simulink model "autotransformerSubtractive"  (R2018a)
settings: Solver=VariableStepAuto  StartTime=0.0  StopTime=0.1  FixedStep=0.01666  RelTol=1e-4
values from neighbouring files (symbols this model uses):
  Freq = 60    [Autotransformer.m]    (also in transformer2wind.m; transformer3wind.m)
  k = 240/2400    (= 0.1)    [Autotransformer.m]    (also in transformer2wind.m)
  L1 = 0.92/(2*pi*Freq)    (= 0.00244037579408)    [Autotransformer.m]    (also in transformer2wind.m = 0.00119366207319; transformer3wind.m = 0.00119366207319)
  L2 = 0.009/(2*pi*Freq)    (= 2.38732414638e-05)    [Autotransformer.m]    (also in transformer2wind.m = 1.19366207319e-05; transformer3wind.m = 1.19366207319e-05)
  Ll = Xl/(2*pi*Freq)    (= 0.0202328075769)    [Autotransformer.m]    (also in transformer2wind.m = 0.000610160156975)
  Lo = 4370/(2*pi*Freq)    (= 11.5917850219)    [Autotransformer.m]    (also in transformer2wind.m = 4.11150269654; transformer3wind.m = 4.11150269654)
  R1 = 0.72    [Autotransformer.m]    (also in transformer2wind.m = 0.2; transformer3wind.m = 0.2)
  R2 = 0.007    [Autotransformer.m]    (also in transformer2wind.m = 0.002; transformer3wind.m = 0.002)
  Rl = 440000/(208*208)    (= 10.1701183432)    [Autotransformer.m]    (also in transformer2wind.m = 0.307480832)
  Ro = 632    [Autotransformer.m]    (also in transformer2wind.m = 10000; transformer3wind.m = 10000)
  S = 50000    [Autotransformer.m]    (also in transformer2wind.m = 150000; transformer3wind.m = 150000)
  V1 = 2400    [Autotransformer.m]    (also in transformer3wind.m)
  V2 = 240    [Autotransformer.m]    (also in transformer2wind.m; transformer3wind.m)
  Vs = 2405*sqrt(2)    [Autotransformer.m]    (also in transformer2wind.m = 2455*sqrt(2); transformer3wind.m = 2455*sqrt(2))
libraries: fl_lib x15, powerlib x9, nesl_utility x5
settings Model: Creator=Noor  LastModifiedBy=Noor

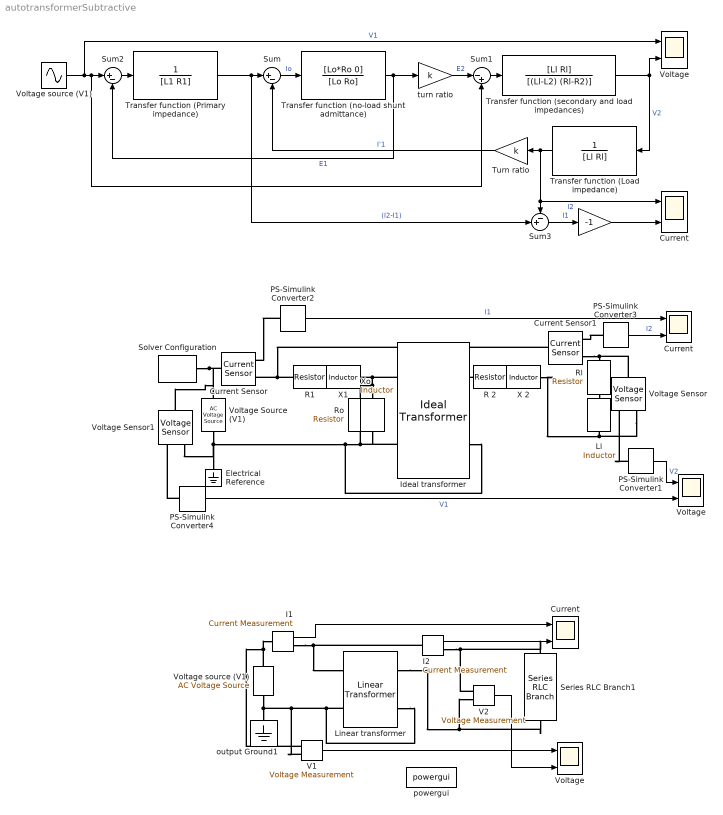
== system autotransformerSubtractive ==
  "  " : Gain  Gain=-1
  " Current" : Scope  NumInputPorts=2
  " Voltage" : Scope  NumInputPorts=2
  Current : Scope  NumInputPorts=2
  "Current " : Scope  NumInputPorts=2
  Current Sensor : fl_lib/Electrical/Electrical Sensors/Current Sensor
  Current Sensor1 : fl_lib/Electrical/Electrical Sensors/Current Sensor
  Electrical Reference : fl_lib/Electrical/Electrical Elements/Electrical Reference
  "I1 " : powerlib/Measurements/Current Measurement  Tag=PoWeRsYsTeMmEaSuReMeNt  PhasorSimulation=off  OutputType=Magnitude  PSBequivalent=0
  "I2 " : powerlib/Measurements/Current Measurement  Tag=PoWeRsYsTeMmEaSuReMeNt  PhasorSimulation=off  OutputType=Magnitude  PSBequivalent=0
  Ideal transformer : fl_lib/Electrical/Electrical Elements/Ideal Transformer  n=1/k  i1_specify=off  i1_priority=None  i1=0 A  i1_nominal_specify=off  i1_nominal_unit=A  i1_nominal_value=1  v1_specify=off  v1_priority=None  v1=0 V  v1_nominal_specify=off  v1_nominal_unit=V  v1_nominal_value=1  i2_specify=off  i2_priority=None  i2=0 A  i2_nominal_specify=off  i2_nominal_unit=A  i2_nominal_value=1  v2_specify=off  v2_priority=None  v2=0 V  v2_nominal_specify=off  v2_nominal_unit=V  v2_nominal_value=1
      settings: SourceProductName=Simscape  SourceProductBaseCode=SS
  Linear transformer : powerlib/Elements/Linear Transformer  UNITS=SI  NominalPower=[S Freq]  winding1=[V1 R1 L1]  winding2=[V2 R2 L2]  ThreeWindings=off  winding3=[3.15e+05 0.7938 0.084225]  RmLm=[Ro Lo]  Measurements=None  DataType=on
  Ll : fl_lib/Electrical/Electrical Elements/Inductor  l=Ll H  r=0 Ohm  g=0 1/Ohm  i_specify=off  i_priority=None  i=0 A  i_nominal_specify=off  i_nominal_unit=A  i_nominal_value=1  v_specify=off  v_priority=None  v=0 V  v_nominal_specify=off  v_nominal_unit=V  v_nominal_value=1  i_L_specify=off  i_L_priority=High  i_L=0 A  i_L_nominal_specify=off  i_L_nominal_unit=A  i_L_nominal_value=1
  PS-Simulink Converter{1..4} (4 alike) : nesl_utility/PS-Simulink Converter  PhysicalDomain=network_engine_domain  SubClassName=ps_output  LeftPortType=input  RightPortType=output  PseudoPeriodic=off  Frequencies=[]  Unit=1  AffineConversion=off
  R 2 : fl_lib/Electrical/Electrical Elements/Resistor  R=R2 Ohm  i_specify=off  i_priority=None  i=0 A  i_nominal_specify=off  i_nominal_unit=A  i_nominal_value=1  v_specify=off  v_priority=None  v=0 V  v_nominal_specify=off  v_nominal_unit=V  v_nominal_value=1
  R1 : fl_lib/Electrical/Electrical Elements/Resistor  R=R1 Ohm  i_specify=off  i_priority=None  i=0 A  i_nominal_specify=off  i_nominal_unit=A  i_nominal_value=1  v_specify=off  v_priority=None  v=0 V  v_nominal_specify=off  v_nominal_unit=V  v_nominal_value=1
  Rl : fl_lib/Electrical/Electrical Elements/Resistor  R=Rl Ohm  i_specify=off  i_priority=None  i=0 A  i_nominal_specify=off  i_nominal_unit=A  i_nominal_value=1  v_specify=off  v_priority=None  v=0 V  v_nominal_specify=off  v_nominal_unit=V  v_nominal_value=1
  Ro : fl_lib/Electrical/Electrical Elements/Resistor  R=Ro Ohm  i_specify=off  i_priority=None  i=0 A  i_nominal_specify=off  i_nominal_unit=A  i_nominal_value=1  v_specify=off  v_priority=None  v=0 V  v_nominal_specify=off  v_nominal_unit=V  v_nominal_value=1
  Series RLC Branch1 : powerlib/Elements/Series RLC Branch  LConnTagsString=__new0  RConnTagsString=__new0  BranchType=RL  Resistance=Rl  Inductance=Ll  SetiL0=off  InitialCurrent=0  Capacitance=1e-6  Setx0=off  InitialVoltage=0  Measurements=None
  Solver Configuration : nesl_utility/Solver Configuration  PhysicalDomain=network_engine_domain  SubClassName=solver  LeftPortType=input  RightPortType=generic  Tones=[]  Harmonics=[]  SimulateNoise=off  Profile=off  UseLocalSampling=off  EnableSwitchedLinearOptims=on  FrequencyDomain=off  UseCCode=off  RelTol=0.001  AbsTol=1e-06  MinStep=1e-09  ToWorkspace=off  RevertToSquareIcSolve=off  NumHomotopyIterations=100  PhasorMode=off  PhasorModeNumHarmonics=1  DoDC=off  ResidualTolerance=1e-09  UseLocalSolver=off  LocalSolverChoice=NE_BACKWARD_EULER_ADVANCER  LocalSolverSampleTime=0.001  DoFixedCost=off  MaxNonlinIter=3  MaxModeIter=2  LinearAlgebra=Sparse  EquationFormulation=NE_TIME_EF  DelaysMemoryBudget=1024  AutomaticFiltering=on  FilteringTimeConstant=0.001
  Sum : Sum  Inputs=|+-
  Sum1 : Sum  Inputs=|-+
  Sum2 : Sum  Inputs=|+-
  Sum3 : Sum  Inputs=-+|
  Transfer function (Load impedance) : TransferFcn  Denominator=[Ll Rl]
  "Transfer function (Primary impedance) " : TransferFcn  Denominator=[L1 R1]
  Transfer function (no-load shunt admittance) : TransferFcn  Numerator=[Lo*Ro 0]  Denominator=[Lo Ro]
  Transfer function (secondary and load impedances) : TransferFcn  Numerator=[Ll Rl]  Denominator=[(Ll-L2) (Rl-R2)]
  Turn ratio : Gain  Gain=k
  V1 : powerlib/Measurements/Voltage Measurement  Tag=PoWeRsYsTeMmEaSuReMeNt  PhasorSimulation=off  OutputType=Magnitude  PSBequivalent=0
  V2 : powerlib/Measurements/Voltage Measurement  Tag=PoWeRsYsTeMmEaSuReMeNt  PhasorSimulation=off  OutputType=Magnitude  PSBequivalent=0
  Voltage : Scope  NumInputPorts=2
  Voltage source (V1) : powerlib/Electrical Sources/AC Voltage Source  Amplitude=Vs  Phase=0  Frequency=Freq  SampleTime=0  Measurements=None  BusType=swing  Pref=10e3  Qref=0  Qmin=-inf  Qmax=+inf
  "Voltage  " : Scope  NumInputPorts=2
  Voltage Sensor : fl_lib/Electrical/Electrical Sensors/Voltage Sensor
  Voltage Sensor1 : fl_lib/Electrical/Electrical Sensors/Voltage Sensor
  Voltage Source (V1) : fl_lib/Electrical/Electrical Sources/AC Voltage Source  amp=Vs V  shift=0 deg  frequency=Freq Hz  omega=0 rad/s
  "Voltage source (V1) " : Sin  Amplitude=Vs  Frequency=2*pi*Freq  SampleTime=0
  X 2 : fl_lib/Electrical/Electrical Elements/Inductor  l=L2 H  r=0 Ohm  g=0 1/Ohm  i_specify=off  i_priority=None  i=0 A  i_nominal_specify=off  i_nominal_unit=A  i_nominal_value=1  v_specify=off  v_priority=None  v=0 V  v_nominal_specify=off  v_nominal_unit=V  v_nominal_value=1  i_L_specify=off  i_L_priority=High  i_L=0 A  i_L_nominal_specify=off  i_L_nominal_unit=A  i_L_nominal_value=1
  X1 : fl_lib/Electrical/Electrical Elements/Inductor  l=L1 H  r=0 Ohm  g=0 1/Ohm  i_specify=off  i_priority=None  i=0 A  i_nominal_specify=off  i_nominal_unit=A  i_nominal_value=1  v_specify=off  v_priority=None  v=0 V  v_nominal_specify=off  v_nominal_unit=V  v_nominal_value=1  i_L_specify=off  i_L_priority=High  i_L=0 A  i_L_nominal_specify=off  i_L_nominal_unit=A  i_L_nominal_value=1
  Xo : fl_lib/Electrical/Electrical Elements/Inductor  l=Lo H  r=0 Ohm  g=0 1/Ohm  i_specify=off  i_priority=None  i=0 A  i_nominal_specify=off  i_nominal_unit=A  i_nominal_value=1  v_specify=off  v_priority=None  v=0 V  v_nominal_specify=off  v_nominal_unit=V  v_nominal_value=1  i_L_specify=off  i_L_priority=High  i_L=0 A  i_L_nominal_specify=off  i_L_nominal_unit=A  i_L_nominal_value=1
  output Ground1 : powerlib/Elements/Ground  LConnTagsString=a
  powergui : powerlib/powergui  SimulationMode=Continuous  SampleTime=0  frequency=60  Iterations=50  frequencyindice=60  Pbase=100e6  ErrMax=1e-4  UnitsV=kV  UnitsW=MW  buscounter=0  FunctionMessages=off  echomessages=off  EnableUseOfTLC=off  CurrentSourceSwitches=off  DisableSnubberDevices=off  DisableRonSwitches=off  DisableVfSwitches=off  DisplayEquations=off  SolverType=Tustin/Backward Euler (TBE)  Interpol=off  ExternalGateDelay=off  methode=off  Ts=100  x0status=blocks  SPID=off  SwTol=0  HookPort=off  RestoreLinks=warning  ResistiveCurrentMeasurement=off  Frange=[0:2:500]  Ylog=off  Xlog=on  ShowGrid=off  save=off  variable=ZData  structure=0  ZoomFFT=on  StartTime=0.0  cycles=1  DisplayStyle=1  fundamental=60  FreqAxis=off  MaxFrequency=1000  frequencyindicesteady=1  RmsSteady=1  display=off
  turn ratio : Gain  Gain=k
  wires:
  PS-Simulink Converter1/1 -> Voltage/1  "V2"
  Transfer function (Load impedance)/1 -> Current/1, Sum3/1, Turn ratio/1  "I2"
  turn ratio/1 -> Sum1/1  "E2"
  Transfer function (secondary and load impedances)/1 -> "Voltage  "/2, Transfer function (Load impedance)/1  "V2"
  Sum2/1 -> "Transfer function (Primary impedance) "/1
  "Voltage source (V1) "/1 -> "Voltage  "/1, Sum2/1, Sum1/2  "V1"
  Transfer function (no-load shunt admittance)/1 -> turn ratio/1, Sum2/2  "E1"
  Turn ratio/1 -> Sum/2  "I'1"
  Sum/1 -> Transfer function (no-load shunt admittance)/1  "Io"
  Sum1/1 -> Transfer function (secondary and load impedances)/1
  "Transfer function (Primary impedance) "/1 -> Sum3/2, Sum/1  "(I2-I1)"
  Sum3/1 -> "  "/1  "I1"
  PS-Simulink Converter3/1 -> "Current "/2  "I2"
  PS-Simulink Converter2/1 -> "Current "/1  "I1"
  PS-Simulink Converter4/1 -> Voltage/2  "V1"
  "I2 "/1 -> " Current"/2
  "I1 "/1 -> " Current"/1
  V2/1 -> " Voltage"/2
  V1/1 -> " Voltage"/1
  "  "/1 -> Current/2
  connections:
  R1/RConn1 -- X1/LConn1
  X 2/LConn1 -- R 2/RConn1
  Rl/RConn1 -- Ll/LConn1
  Voltage Sensor/LConn1 -- Current Sensor1/RConn2 -- Rl/LConn1
  Ro/LConn1 -- Xo/LConn1 -- Ideal transformer/LConn1 -- X1/RConn1
  Solver Configuration/RConn1 -- Current Sensor/LConn1 -- Voltage Sensor1/LConn1 -- Voltage Source (V1)/LConn1
  PS-Simulink Converter2/LConn1 -- Current Sensor/RConn1
  PS-Simulink Converter3/LConn1 -- Current Sensor1/RConn1
  PS-Simulink Converter1/LConn1 -- Voltage Sensor/RConn1
  R1/LConn1 -- Current Sensor1/LConn1 -- Current Sensor/RConn2
  V2/LConn1 -- Series RLC Branch1/LConn1 -- "I2 "/RConn1
  Electrical Reference/LConn1 -- Voltage Sensor1/RConn2 -- Voltage Source (V1)/RConn1 -- Ideal transformer/RConn2 -- Ideal transformer/LConn2 -- Xo/RConn1 -- Ro/RConn1
  "I1 "/RConn1 -- "I2 "/LConn1 -- Linear transformer/LConn1
  Linear transformer/LConn2 -- Linear transformer/RConn2 -- V1/LConn2 -- output Ground1/LConn1 -- Voltage source (V1)/LConn1
  Voltage source (V1)/RConn1 -- V1/LConn1 -- "I1 "/LConn1
  PS-Simulink Converter4/LConn1 -- Voltage Sensor1/RConn1
  Voltage Sensor/RConn2 -- X 2/RConn1 -- Ll/RConn1
  R 2/LConn1 -- Ideal transformer/RConn1
  Series RLC Branch1/RConn1 -- V2/LConn2 -- Linear transformer/RConn1
